simulink model "SF043A_TqOscn"  (R2013b)
settings: Solver=FixedStepDiscrete  SolverMode=SingleTasking  StartTime=0.0  StopTime=1  FixedStep=0.002  RelTol=1e-3
values from neighbouring files (symbols this model uses):
  ARCHGLBPRM_2MILLISEC_SEC_F32 = DataDict.Constant    [SF043A_TqOscn_DataDict.m]
  ARCHGLBPRM_2PI_ULS_F32 = DataDict.Constant    [SF043A_TqOscn_DataDict.m]
  DCTHD_MOTNWTMTR_F32 = DataDict.Constant    [SF043A_TqOscn_DataDict.m]
  DFTFALLRAMPRATE_MOTNWTMTRPERSEC_F32 = DataDict.Constant    [SF043A_TqOscn_DataDict.m]
  DFTPHAAGINC_MATRAD_F32 = DataDict.Constant    [SF043A_TqOscn_DataDict.m]
  DFTRISNGRAMPRATE_MOTNWTMTRPERSEC_F32 = DataDict.Constant    [SF043A_TqOscn_DataDict.m]
  FltInj_f32 = DataDict.Client    [SF043A_TqOscn_DataDict.m]
  FLTINJ_TQOSCN_PREFINALCMD = DataDict.Constant    [SF043A_TqOscn_DataDict.m]
  MAXAMP_MOTNWTMTR_F32 = DataDict.Constant    [SF043A_TqOscn_DataDict.m]
  MAXRAMPRATE_MOTNWTMTR_F32 = DataDict.Constant    [SF043A_TqOscn_DataDict.m]
  MINAMP_MOTNWTMTR_F32 = DataDict.Constant    [SF043A_TqOscn_DataDict.m]
  MINRAMPRATE_MOTNWTMTR_F32 = DataDict.Constant    [SF043A_TqOscn_DataDict.m]
  TqOscnAmpLimY = DataDict.Calibration    [SF043A_TqOscn_DataDict.m]
  TqOscnFallRampRateCal = DataDict.Calibration    [SF043A_TqOscn_DataDict.m]
  TqOscnFrqIn = DataDict.Calibration    [SF043A_TqOscn_DataDict.m]
  TqOscnRisngRampRateCal = DataDict.Calibration    [SF043A_TqOscn_DataDict.m]
  TqOscnUseRampRateCal = DataDict.Calibration    [SF043A_TqOscn_DataDict.m]
libraries: NxtrLim x6, simulink x3, NxtrAbslt x3, Fil x2, FixdToFloat x2, autosarlib x1, NxtrMath x1, FloatToFixd x1
(part 2 of 2)

== system SF043A_TqOscn/TqOscn/TqOscnPer1/Amplitude Rate Limiter/SetToZero ==
  Action Port : ActionPort  ActionType=then
  Constant4 : Constant  Value=0  OutDataTypeStr=single
      settings: AttributesFormatString=%<OutDataTypeStr>
  CopyRight2 : Subsystem  Description=|  mask(Copyright Information){none=on}
      | Copyright info block.                                               
      |                                                                     
      | Place copyright information at the top of every subsystem in design.
      mask prompts: none "No parameters"
      mask help: Place copyright information at the top of every subsystem in design.
      mask Display:
      | NxtrConf = 'Nexteer Confidential';
      | 
      | sys = bdroot; %handle for the current model ("system")
      | first = get_param(sys,'Created');
      | if(isempty(first))
      |     first = datestr(now,'yyyy');
      | else
      |     first = first(end-3:end);  %year is last four digits
      | end
      | 
      | last = get_param(sys,'LastModifiedDate');
      | if isempty(last)
      |     last = datestr(now,'yyyy');
      | else
      |     last = last(end-3:end);
      | end
      | 
      | if strcmp(first,last)
      |     fprintf('%s -- Copyright %s Nexteer',NxtrConf,first)
      | else
      |     fprintf('%s -- %s%s- %s Nexteer',NxtrConf,char(169),first,last)
      | end
  Out1 : Outport
  wires:
  Constant4/1 -> Out1/1

== system SF043A_TqOscn/TqOscn/TqOscnPer1/Amplitude Rate Limiter/UseCals ==
  Action Port : ActionPort  ActionType=then
  Constant1 : Constant  Value=TqOscnRisngRampRateCal
  Constant2 : Constant  Value=TqOscnFallRampRateCal
  CopyRight2 : Subsystem  Description=|  mask(Copyright Information){none=on}
      | Copyright info block.                                               
      |                                                                     
      | Place copyright information at the top of every subsystem in design.
      mask prompts: none "No parameters"
      mask help: Place copyright information at the top of every subsystem in design.
      mask Display:
      | NxtrConf = 'Nexteer Confidential';
      | 
      | sys = bdroot; %handle for the current model ("system")
      | first = get_param(sys,'Created');
      | if(isempty(first))
      |     first = datestr(now,'yyyy');
      | else
      |     first = first(end-3:end);  %year is last four digits
      | end
      | 
      | last = get_param(sys,'LastModifiedDate');
      | if isempty(last)
      |     last = datestr(now,'yyyy');
      | else
      |     last = last(end-3:end);
      | end
      | 
      | if strcmp(first,last)
      |     fprintf('%s -- Copyright %s Nexteer',NxtrConf,first)
      | else
      |     fprintf('%s -- %s%s- %s Nexteer',NxtrConf,char(169),first,last)
      | end
  Out1 : Outport
  Out2 : Outport  Port=2
  wires:
  Constant2/1 -> Out1/1
  Constant1/1 -> Out2/1

== system SF043A_TqOscn/TqOscn/TqOscnPer1/Amplitude Rate Limiter/UseCmd ==
  In1 : Inport
  Action Port : ActionPort  ActionType=else
  Out1 : Outport
  wires:
  In1/1 -> Out1/1

== system SF043A_TqOscn/TqOscn/TqOscnPer1/Amplitude Rate Limiter/UseInputs ==
  In1 : Inport
  In2 : Inport  Port=2
  Action Port : ActionPort  ActionType=else
  Out1 : Outport
  Out2 : Outport  Port=2
  wires:
  In2/1 -> Out2/1
  In1/1 -> Out1/1

== system SF043A_TqOscn/TqOscn/TqOscnPer1/Angle Wrapper/CopyRight2 ==

== system SF043A_TqOscn/TqOscn/TqOscnPer1/Angle Wrapper/Pass_through ==
  In1 : Inport
  Action Port : ActionPort  ActionType=else
  CopyRight2 : Subsystem  Description=|  mask(Copyright Information){none=on}
      | Copyright info block.                                               
      |                                                                     
      | Place copyright information at the top of every subsystem in design.
      mask prompts: none "No parameters"
      mask help: Place copyright information at the top of every subsystem in design.
      mask Display:
      | NxtrConf = 'Nexteer Confidential';
      | 
      | sys = bdroot; %handle for the current model ("system")
      | first = get_param(sys,'Created');
      | if(isempty(first))
      |     first = datestr(now,'yyyy');
      | else
      |     first = first(end-3:end);  %year is last four digits
      | end
      | 
      | last = get_param(sys,'LastModifiedDate');
      | if isempty(last)
      |     last = datestr(now,'yyyy');
      | else
      |     last = last(end-3:end);
      | end
      | 
      | if strcmp(first,last)
      |     fprintf('%s -- Copyright %s Nexteer',NxtrConf,first)
      | else
      |     fprintf('%s -- %s%s- %s Nexteer',NxtrConf,char(169),first,last)
      | end
  Out1 : Outport
  wires:
  In1/1 -> Out1/1

== system SF043A_TqOscn/TqOscn/TqOscnPer1/Angle Wrapper/Subtract_2pi ==
  In1 : Inport
  Action Port : ActionPort  ActionType=then
  Constant : Constant  Value=ARCHGLBPRM_2PI_ULS_F32
  CopyRight2 : Subsystem  Description=|  mask(Copyright Information){none=on}
      | Copyright info block.                                               
      |                                                                     
      | Place copyright information at the top of every subsystem in design.
      mask prompts: none "No parameters"
      mask help: Place copyright information at the top of every subsystem in design.
      mask Display:
      | NxtrConf = 'Nexteer Confidential';
      | 
      | sys = bdroot; %handle for the current model ("system")
      | first = get_param(sys,'Created');
      | if(isempty(first))
      |     first = datestr(now,'yyyy');
      | else
      |     first = first(end-3:end);  %year is last four digits
      | end
      | 
      | last = get_param(sys,'LastModifiedDate');
      | if isempty(last)
      |     last = datestr(now,'yyyy');
      | else
      |     last = last(end-3:end);
      | end
      | 
      | if strcmp(first,last)
      |     fprintf('%s -- Copyright %s Nexteer',NxtrConf,first)
      | else
      |     fprintf('%s -- %s%s- %s Nexteer',NxtrConf,char(169),first,last)
      | end
  Subtract : Sum  Inputs=+-
  Out1 : Outport
  wires:
  In1/1 -> Subtract/1
  Subtract/1 -> Out1/1
  Constant/1 -> Subtract/2

== system SF043A_TqOscn/TqOscn/TqOscnPer1/CheckFlag/CopyRight2 ==

== system SF043A_TqOscn/TqOscn/TqOscnPer1/CheckFlag/SetToZero ==
  Action Port : ActionPort  ActionType=else
  Constant2 : Constant  Value=0  OutDataTypeStr=single
      settings: AttributesFormatString=%<OutDataTypeStr>
  CopyRight2 : Subsystem  Description=|  mask(Copyright Information){none=on}
      | Copyright info block.                                               
      |                                                                     
      | Place copyright information at the top of every subsystem in design.
      mask prompts: none "No parameters"
      mask help: Place copyright information at the top of every subsystem in design.
      mask Display:
      | NxtrConf = 'Nexteer Confidential';
      | 
      | sys = bdroot; %handle for the current model ("system")
      | first = get_param(sys,'Created');
      | if(isempty(first))
      |     first = datestr(now,'yyyy');
      | else
      |     first = first(end-3:end);  %year is last four digits
      | end
      | 
      | last = get_param(sys,'LastModifiedDate');
      | if isempty(last)
      |     last = datestr(now,'yyyy');
      | else
      |     last = last(end-3:end);
      | end
      | 
      | if strcmp(first,last)
      |     fprintf('%s -- Copyright %s Nexteer',NxtrConf,first)
      | else
      |     fprintf('%s -- %s%s- %s Nexteer',NxtrConf,char(169),first,last)
      | end
  Out1 : Outport
  wires:
  Constant2/1 -> Out1/1

== system SF043A_TqOscn/TqOscn/TqOscnPer1/CheckFlag/UseInput ==
  In1 : Inport
  Action Port : ActionPort  ActionType=then
  CopyRight2 : Subsystem  Description=|  mask(Copyright Information){none=on}
      | Copyright info block.                                               
      |                                                                     
      | Place copyright information at the top of every subsystem in design.
      mask prompts: none "No parameters"
      mask help: Place copyright information at the top of every subsystem in design.
      mask Display:
      | NxtrConf = 'Nexteer Confidential';
      | 
      | sys = bdroot; %handle for the current model ("system")
      | first = get_param(sys,'Created');
      | if(isempty(first))
      |     first = datestr(now,'yyyy');
      | else
      |     first = first(end-3:end);  %year is last four digits
      | end
      | 
      | last = get_param(sys,'LastModifiedDate');
      | if isempty(last)
      |     last = datestr(now,'yyyy');
      | else
      |     last = last(end-3:end);
      | end
      | 
      | if strcmp(first,last)
      |     fprintf('%s -- Copyright %s Nexteer',NxtrConf,first)
      | else
      |     fprintf('%s -- %s%s- %s Nexteer',NxtrConf,char(169),first,last)
      | end
  Out1 : Outport
  wires:
  In1/1 -> Out1/1

== system SF043A_TqOscn/TqOscn/TqOscnPer1/DC Check/CopyRight2 ==

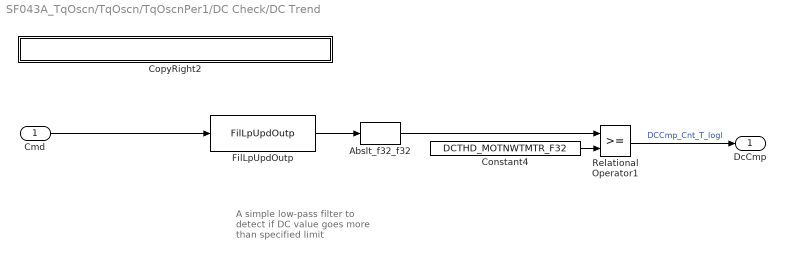
== system SF043A_TqOscn/TqOscn/TqOscnPer1/DC Check/DC Trend ==
  note: A simple low-pass filter to detect if DC value goes more than specified limit
  Cmd : Inport
  Abslt_f32_f32 : NxtrAbslt/Abslt_f32_f32  SFunctionSpec=single y1 = Abslt_f32_f32(single u1)
      settings: AttributesFormatString=%<Name>
  Constant4 : Constant  RequirementInfo={'linktype_rmi_doors' '0000a558 (/E-STEER Core/SubSystem Specifications/Application Functions/SF043A Torque Oscillation)' '#SF043A_335' 'true' 'REQ:SF043A_335' '' } %GIDa_6c203f5b_5b38_493c_a4ae_d80a5c53087b  Value=DCTHD_MOTNWTMTR_F32
  CopyRight2 : Subsystem  Description=|  mask(Copyright Information){none=on}
      | Copyright info block.                                               
      |                                                                     
      | Place copyright information at the top of every subsystem in design.
      mask prompts: none "No parameters"
      mask help: Place copyright information at the top of every subsystem in design.
      mask Display:
      | NxtrConf = 'Nexteer Confidential';
      | 
      | sys = bdroot; %handle for the current model ("system")
      | first = get_param(sys,'Created');
      | if(isempty(first))
      |     first = datestr(now,'yyyy');
      | else
      |     first = first(end-3:end);  %year is last four digits
      | end
      | 
      | last = get_param(sys,'LastModifiedDate');
      | if isempty(last)
      |     last = datestr(now,'yyyy');
      | else
      |     last = last(end-3:end);
      | end
      | 
      | if strcmp(first,last)
      |     fprintf('%s -- Copyright %s Nexteer',NxtrConf,first)
      | else
      |     fprintf('%s -- %s%s- %s Nexteer',NxtrConf,char(169),first,last)
      | end
  FilLpUpdOutp : Fil/FilLpUpdOutp  RequirementInfo={'linktype_rmi_doors' '0000a558 (/E-STEER Core/SubSystem Specifications/Application Functions/SF043A Torque Oscillation)' '#SF043A_334' 'true' 'REQ:SF043A_334' '' } %GIDa_7480e813_7b8e_4b56_a323_4ea049146c63  StVar=PreFinalCmdLpFil
      settings: AttributesFormatString=StVar: %<StVar>
  Relational Operator1 : RelationalOperator  RequirementInfo={'linktype_rmi_doors' '0000a558 (/E-STEER Core/SubSystem Specifications/Application Functions/SF043A Torque Oscillation)' '#SF043A_335' 'true' 'REQ:SF043A_335' '' } %GIDa_618fbe93_81fb_4f23_8b51_b3d5bed42e02  OutDataTypeStr=boolean
  DcCmp : Outport  RequirementInfo={'linktype_rmi_doors' '0000a558 (/E-STEER Core/SubSystem Specifications/Application Functions/SF043A Torque Oscillation)' '#SF043A_335' 'true' 'REQ:SF043A_335' '' } %GIDa_1afcdcae_25d3_461d_aaa1_98d84ed6aaf2
  wires:
  FilLpUpdOutp/1 -> Abslt_f32_f32/1
  Constant4/1 -> Relational Operator1/2
  Relational Operator1/1 -> DcCmp/1  "DCCmp_Cnt_T_logl"
  Abslt_f32_f32/1 -> Relational Operator1/1
  Cmd/1 -> FilLpUpdOutp/1

== system SF043A_TqOscn/TqOscn/TqOscnPer1/DC Check/DC_Detd ==
  Action Port : ActionPort  ActionType=then
  Constant : Constant  Value=0  OutDataTypeStr=single
      settings: AttributesFormatString=%<OutDataTypeStr>
  Constant1 : Constant  Value=true  OutDataTypeStr=boolean
      settings: AttributesFormatString=%<OutDataTypeStr>
  CopyRight2 : Subsystem  Description=|  mask(Copyright Information){none=on}
      | Copyright info block.                                               
      |                                                                     
      | Place copyright information at the top of every subsystem in design.
      mask prompts: none "No parameters"
      mask help: Place copyright information at the top of every subsystem in design.
      mask Display:
      | NxtrConf = 'Nexteer Confidential';
      | 
      | sys = bdroot; %handle for the current model ("system")
      | first = get_param(sys,'Created');
      | if(isempty(first))
      |     first = datestr(now,'yyyy');
      | else
      |     first = first(end-3:end);  %year is last four digits
      | end
      | 
      | last = get_param(sys,'LastModifiedDate');
      | if isempty(last)
      |     last = datestr(now,'yyyy');
      | else
      |     last = last(end-3:end);
      | end
      | 
      | if strcmp(first,last)
      |     fprintf('%s -- Copyright %s Nexteer',NxtrConf,first)
      | else
      |     fprintf('%s -- %s%s- %s Nexteer',NxtrConf,char(169),first,last)
      | end
  Cmd : Outport
  Excdd : Outport  Port=2
  wires:
  Constant/1 -> Cmd/1
  Constant1/1 -> Excdd/1

== system SF043A_TqOscn/TqOscn/TqOscnPer1/DC Check/DC_ok ==
  In1 : Inport
  Action Port : ActionPort  ActionType=else
  Constant1 : Constant  Value=false  OutDataTypeStr=boolean
      settings: AttributesFormatString=%<OutDataTypeStr>
  CopyRight2 : Subsystem  Description=|  mask(Copyright Information){none=on}
      | Copyright info block.                                               
      |                                                                     
      | Place copyright information at the top of every subsystem in design.
      mask prompts: none "No parameters"
      mask help: Place copyright information at the top of every subsystem in design.
      mask Display:
      | NxtrConf = 'Nexteer Confidential';
      | 
      | sys = bdroot; %handle for the current model ("system")
      | first = get_param(sys,'Created');
      | if(isempty(first))
      |     first = datestr(now,'yyyy');
      | else
      |     first = first(end-3:end);  %year is last four digits
      | end
      | 
      | last = get_param(sys,'LastModifiedDate');
      | if isempty(last)
      |     last = datestr(now,'yyyy');
      | else
      |     last = last(end-3:end);
      | end
      | 
      | if strcmp(first,last)
      |     fprintf('%s -- Copyright %s Nexteer',NxtrConf,first)
      | else
      |     fprintf('%s -- %s%s- %s Nexteer',NxtrConf,char(169),first,last)
      | end
  Cmd : Outport
  Excdd : Outport  Port=2
  wires:
  In1/1 -> Cmd/1
  Constant1/1 -> Excdd/1

== system SF043A_TqOscn/TqOscn/TqOscnPer1/FltInj_f32 client/CodeGen ==
  note: NOTE 1:  Simulink 2013b cannot handle InOut arguments, so the operation
      |                 prototype inside this block is not quite right.
      |
      | NOTE 2:  Do not use this variant for simulation.  Sig_Out = zero, always.
  note: FltInj_f32(float32 *SigPah, uint16 LocnKey)
  Sig : Inport
  "LocnKey  " : Inport  Port=2
  CopyRight1 : Subsystem  Description=|  mask(Copyright Information){none=on}
      | Copyright info block.                                               
      |                                                                     
      | Place copyright information at the top of every subsystem in design.
      mask prompts: none "No parameters"
      mask help: Place copyright information at the top of every subsystem in design.
      mask Display:
      | NxtrConf = 'Nexteer Confidential';
      | 
      | sys = bdroot; %handle for the current model ("system")
      | first = get_param(sys,'Created');
      | if(isempty(first))
      |     first = datestr(now,'yyyy');
      | else
      |     first = first(end-3:end);  %year is last four digits
      | end
      | 
      | last = get_param(sys,'LastModifiedDate');
      | if isempty(last)
      |     last = datestr(now,'yyyy');
      | else
      |     last = last(end-3:end);
      | end
      | 
      | if strcmp(first,last)
      |     fprintf('%s -- Copyright %s Nexteer',NxtrConf,first)
      | else
      |     fprintf('%s -- %s%s- %s Nexteer',NxtrConf,char(169),first,last)
      | end
  Invoke AUTOSAR Server Operation : autosarlib/Invoke AUTOSAR Server Operation  portName=FltInj_f32  operationPrototype=FltInj_f32(IN single SigPah_ArgIn, OUT single SigPah_ArgOut, IN uint16 LocnKey)  interfacePath=/AUTOSAR/Interface  serverType=Application software  showErrorStatus=off  SAMPLETIME=-1  showARPortLabels=on
  Sig_Out : Outport  OutDataTypeStr=single
  wires:
  Sig/1 -> Invoke AUTOSAR Server Operation/1
  "LocnKey  "/1 -> Invoke AUTOSAR Server Operation/2
  Invoke AUTOSAR Server Operation/1 -> Sig_Out/1

== system SF043A_TqOscn/TqOscn/TqOscnPer1/FltInj_f32 client/CopyRight1 ==

== system SF043A_TqOscn/TqOscn/TqOscnPer1/FltInj_f32 client/Sim ==
  note: This block requires no modification by FDD author.
      |
      | This block does not actually simulate any fault injection.  It is simply a pass-thru.
      |
      | Input port (#2) simply terminates its signal, but we are trying to force the FDD author
      | to properly use the FltInjectionLocType enumeration in FDD model.
  note: EA4.x Fault Injection
  Sig : Inport
  "LocnKey  " : Inport  Port=2  OutDataTypeStr=uint16
  CopyRight1 : Subsystem  Description=|  mask(Copyright Information){none=on}
      | Copyright info block.                                               
      |                                                                     
      | Place copyright information at the top of every subsystem in design.
      mask prompts: none "No parameters"
      mask help: Place copyright information at the top of every subsystem in design.
      mask Display:
      | NxtrConf = 'Nexteer Confidential';
      | 
      | sys = bdroot; %handle for the current model ("system")
      | first = get_param(sys,'Created');
      | if(isempty(first))
      |     first = datestr(now,'yyyy');
      | else
      |     first = first(end-3:end);  %year is last four digits
      | end
      | 
      | last = get_param(sys,'LastModifiedDate');
      | if isempty(last)
      |     last = datestr(now,'yyyy');
      | else
      |     last = last(end-3:end);
      | end
      | 
      | if strcmp(first,last)
      |     fprintf('%s -- Copyright %s Nexteer',NxtrConf,first)
      | else
      |     fprintf('%s -- %s%s- %s Nexteer',NxtrConf,char(169),first,last)
      | end
  Terminator : Terminator
  Sig_Out : Outport
  wires:
  Sig/1 -> Sig_Out/1
  "LocnKey  "/1 -> Terminator/1

== system SF043A_TqOscn/TqOscn/TqOscnPer1/Set_false/CopyRight2 ==

== system SF043A_TqOscn/TqOscn/TqOscnPer1/Set_true/CopyRight2 ==

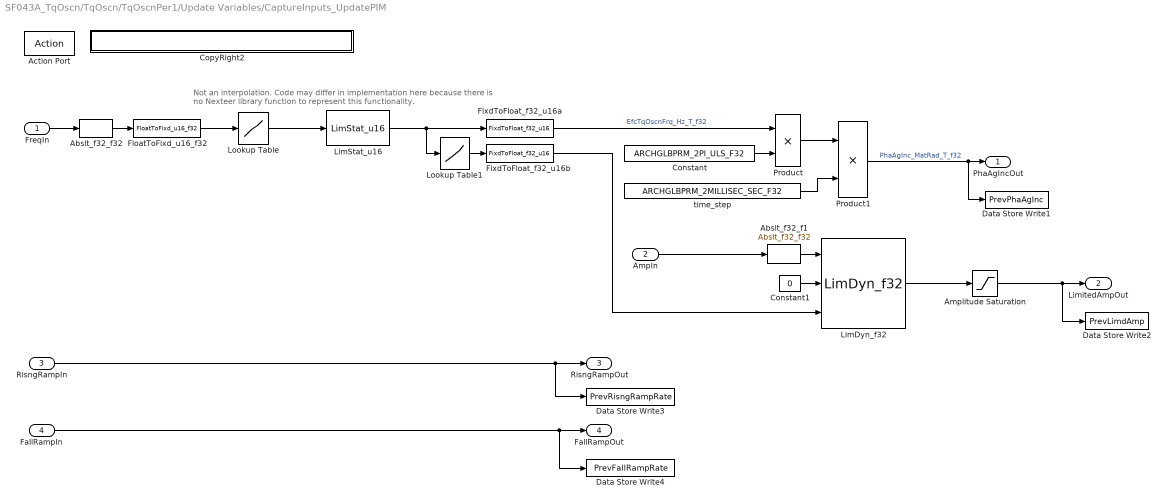
== system SF043A_TqOscn/TqOscn/TqOscnPer1/Update Variables/CaptureInputs_UpdatePIM ==
  note: Not an interpolation.  Code may differ in implementation here because there
      | is no Nexteer library function to represent this functionality.
  FreqIn : Inport  RequirementInfo={} %GIDa_1e1cd702_07fe_49fe_8947_31431a58e45b
  AmpIn : Inport  RequirementInfo={'linktype_rmi_doors' '0000a558 (/E-STEER Core/SubSystem Specifications/Application Functions/SF043A Torque Oscillation)' '#SF043A_320' 'true' 'REQ:SF043A_320' '' } %GIDa_8088d360_8b23_47d1_855a_eb1de7ebd5e4  Port=2
  RisngRampIn : Inport  RequirementInfo={'linktype_rmi_doors' '0000a558 (/E-STEER Core/SubSystem Specifications/Application Functions/SF043A Torque Oscillation)' '#SF043A_321' 'true' 'REQ:SF043A_321' '' } %GIDa_b7d07da4_db6a_4e3d_9af0_8782b4d0f024  Port=3
  FallRampIn : Inport  RequirementInfo={'linktype_rmi_doors' '0000a558 (/E-STEER Core/SubSystem Specifications/Application Functions/SF043A Torque Oscillation)' '#SF043A_322' 'true' 'REQ:SF043A_322' '' } %GIDa_962124a2_4b93_46f5_ace1_33638640915d  Port=4
  Action Port : ActionPort  ActionType=then
  Abslt_f32_f1 : NxtrAbslt/Abslt_f32_f32  RequirementInfo={'linktype_rmi_doors' '0000a558 (/E-STEER Core/SubSystem Specifications/Application Functions/SF043A Torque Oscillation)' '#SF043A_320' 'true' 'REQ:SF043A_320' '' } %GIDa_686dcb48_c1ec_4c2a_924a_e657627dc353  SFunctionSpec=single y1 = Abslt_f32_f32(single u1)
      settings: AttributesFormatString=%<Name>
  Abslt_f32_f32 : NxtrAbslt/Abslt_f32_f32  RequirementInfo={} %GIDa_20961518_0603_4677_bd06_aafd74fe8b47  SFunctionSpec=single y1 = Abslt_f32_f32(single u1)
      settings: AttributesFormatString=%<Name>
  Amplitude Saturation : Saturate  RequirementInfo={'linktype_rmi_doors' '0000a558 (/E-STEER Core/SubSystem Specifications/Application Functions/SF043A Torque Oscillation)' '#SF043A_320' 'true' 'REQ:SF043A_320' '' ; 'linktype_rmi_doors' '0000a558 (/E-STEER Core/SubSystem Specifications/Application Functions/SF043A Torque Oscillation)' '#SF043A_323' 'true' 'REQ:SF043A_323' '' } %GIDa_b14632e0_b3b4_4b21_aab6_08b820319b05  UpperLimit=MAXAMP_MOTNWTMTR_F32  LowerLimit=MINAMP_MOTNWTMTR_F32
      settings: AttributesFormatString=UPR=%<UpperLimit>\nLWR=%<LowerLimit>
  Constant : Constant  Value=ARCHGLBPRM_2PI_ULS_F32
  Constant1 : Constant  RequirementInfo={'linktype_rmi_doors' '0000a558 (/E-STEER Core/SubSystem Specifications/Application Functions/SF043A Torque Oscillation)' '#SF043A_320' 'true' 'REQ:SF043A_320' '' } %GIDa_c355547a_ffc8_4f22_aa5f_e81363987f9d  Value=0  OutDataTypeStr=single
      settings: AttributesFormatString=%<OutDataTypeStr>
  CopyRight2 : Subsystem  Description=|  mask(Copyright Information){none=on}
      | Copyright info block.                                               
      |                                                                     
      | Place copyright information at the top of every subsystem in design.
      mask prompts: none "No parameters"
      mask help: Place copyright information at the top of every subsystem in design.
      mask Display:
      | NxtrConf = 'Nexteer Confidential';
      | 
      | sys = bdroot; %handle for the current model ("system")
      | first = get_param(sys,'Created');
      | if(isempty(first))
      |     first = datestr(now,'yyyy');
      | else
      |     first = first(end-3:end);  %year is last four digits
      | end
      | 
      | last = get_param(sys,'LastModifiedDate');
      | if isempty(last)
      |     last = datestr(now,'yyyy');
      | else
      |     last = last(end-3:end);
      | end
      | 
      | if strcmp(first,last)
      |     fprintf('%s -- Copyright %s Nexteer',NxtrConf,first)
      | else
      |     fprintf('%s -- %s%s- %s Nexteer',NxtrConf,char(169),first,last)
      | end
  Data Store Write1 : DataStoreWrite  DataStoreName=PrevPhaAgInc
  Data Store Write2 : DataStoreWrite  RequirementInfo={'linktype_rmi_doors' '0000a558 (/E-STEER Core/SubSystem Specifications/Application Functions/SF043A Torque Oscillation)' '#SF043A_320' 'true' 'REQ:SF043A_320' '' } %GIDa_684092d3_0e9c_4b10_90ad_6b2ae104cb4a  DataStoreName=PrevLimdAmp
  Data Store Write3 : DataStoreWrite  RequirementInfo={'linktype_rmi_doors' '0000a558 (/E-STEER Core/SubSystem Specifications/Application Functions/SF043A Torque Oscillation)' '#SF043A_321' 'true' 'REQ:SF043A_321' '' } %GIDa_a20425e6_b584_439e_a32a_f492801bed71  DataStoreName=PrevRisngRampRate
  Data Store Write4 : DataStoreWrite  RequirementInfo={'linktype_rmi_doors' '0000a558 (/E-STEER Core/SubSystem Specifications/Application Functions/SF043A Torque Oscillation)' '#SF043A_322' 'true' 'REQ:SF043A_322' '' } %GIDa_8daa8598_b3f2_434a_b3dd_69d33c4d5e6c  DataStoreName=PrevFallRampRate
  FixdToFloat_f32_u16a : FixdToFloat/FixdToFloat_f32_u16  Param1=8
  FixdToFloat_f32_u16b : FixdToFloat/FixdToFloat_f32_u16  Param1=11
  FloatToFixd_u16_f32 : FloatToFixd/FloatToFixd_u16_f32  RequirementInfo={} %GIDa_ab6b0326_8659_495f_9d5e_ae96f25dc97e  Param1=8
  LimDyn_f32 : NxtrLim/LimDyn_f32  RequirementInfo={'linktype_rmi_doors' '0000a558 (/E-STEER Core/SubSystem Specifications/Application Functions/SF043A Torque Oscillation)' '#SF043A_320' 'true' 'REQ:SF043A_320' '' } %GIDa_6df0978f_0905_4878_80b3_8930e7448859
  LimStat_u16 : NxtrLim/LimStat_u16  RequirementInfo={'linktype_rmi_doors' '0000a558 (/E-STEER Core/SubSystem Specifications/Application Functions/SF043A Torque Oscillation)' '#SF043A_315' 'true' 'REQ:SF043A_315' '' } %GIDa_3eeeaba6_26b8_4e57_99e8_6c115ad5e6c8  LoLim=MINFRQ_CNT_U16  HiLim=MAXFRQ_CNT_U16
      settings: AttributesFormatString=|
      | Low Limit: %<LoLim>
      | High Limit:%<HiLim>
  Lookup Table : Lookup  RequirementInfo={'linktype_rmi_doors' '0000a558 (/E-STEER Core/SubSystem Specifications/Application Functions/SF043A Torque Oscillation)' '#SF043A_316' 'true' 'REQ:SF043A_316' '' ; 'linktype_rmi_doors' '0000a558 (/E-STEER Core/SubSystem Specifications/Application Functions/SF043A Torque Oscillation)' '#SF043A_317' 'true' 'REQ:SF043A_317' '' ; 'linktype_rmi_doors' '0000a558 (/E-STEER Core/SubSystem Specifications/Application Functions/SF043A Torque Oscillation)' '#SF043A_318' 'true' 'REQ:SF043A_318' '' } %GIDa_2a87b88c_2148_4626_8153_3d00cbb05ac0  InputValues=TqOscnFrqIn  Table=TqOscnFrqIn  LookUpMeth=Use Input Below
      settings: AttributesFormatString=Input=%<InputValues>\nOutput=%<OutputValues>\nLookup Method=\n%<LookUpMeth>
  Lookup Table1 : Lookup  RequirementInfo={'linktype_rmi_doors' '0000a558 (/E-STEER Core/SubSystem Specifications/Application Functions/SF043A Torque Oscillation)' '#SF043A_324' 'true' 'REQ:SF043A_324' '' } %GIDa_13f9bc77_c553_4d5c_8f17_4791133e4b15  InputValues=TqOscnFrqIn  Table=TqOscnAmpLimY  LookUpMeth=Use Input Below
      settings: AttributesFormatString=Input=%<InputValues>\nOutput=%<OutputValues>\nLookup Method=\n%<LookUpMeth>
  Product : Product  RndMeth=Zero
  Product1 : Product  RndMeth=Zero
  time_step : Constant  Value=ARCHGLBPRM_2MILLISEC_SEC_F32
  PhaAgIncOut : Outport
  LimitedAmpOut : Outport  RequirementInfo={'linktype_rmi_doors' '0000a558 (/E-STEER Core/SubSystem Specifications/Application Functions/SF043A Torque Oscillation)' '#SF043A_320' 'true' 'REQ:SF043A_320' '' } %GIDa_feed8225_5bb0_4298_b6e6_992887f1e478  Port=2
  RisngRampOut : Outport  RequirementInfo={'linktype_rmi_doors' '0000a558 (/E-STEER Core/SubSystem Specifications/Application Functions/SF043A Torque Oscillation)' '#SF043A_321' 'true' 'REQ:SF043A_321' '' } %GIDa_b10902d9_9d3b_44d9_b725_798dc8615d28  Port=3
  FallRampOut : Outport  RequirementInfo={'linktype_rmi_doors' '0000a558 (/E-STEER Core/SubSystem Specifications/Application Functions/SF043A Torque Oscillation)' '#SF043A_322' 'true' 'REQ:SF043A_322' '' } %GIDa_aa2544d0_c17f_4ce5_be5d_55bb8d958bae  Port=4
  wires:
  AmpIn/1 -> Abslt_f32_f1/1
  Lookup Table/1 -> LimStat_u16/1
  LimStat_u16/1 -> FixdToFloat_f32_u16a/1, Lookup Table1/1
  Product/1 -> Product1/1
  time_step/1 -> Product1/2
  LimDyn_f32/1 -> Amplitude Saturation/1
  FreqIn/1 -> Abslt_f32_f32/1
  Lookup Table1/1 -> FixdToFloat_f32_u16b/1
  Constant/1 -> Product/2
  Abslt_f32_f1/1 -> LimDyn_f32/1
  Abslt_f32_f32/1 -> FloatToFixd_u16_f32/1
  Amplitude Saturation/1 -> Data Store Write2/1, LimitedAmpOut/1
  Product1/1 -> Data Store Write1/1, PhaAgIncOut/1  "PhaAgInc_MatRad_T_f32"
  FallRampIn/1 -> Data Store Write4/1, FallRampOut/1
  Constant1/1 -> LimDyn_f32/2
  RisngRampIn/1 -> Data Store Write3/1, RisngRampOut/1
  FloatToFixd_u16_f32/1 -> Lookup Table/1
  FixdToFloat_f32_u16a/1 -> Product/1  "EfcTqOscnFrq_Hz_T_f32"
  FixdToFloat_f32_u16b/1 -> LimDyn_f32/3

== system SF043A_TqOscn/TqOscn/TqOscnPer1/Update Variables/CopyRight2 ==

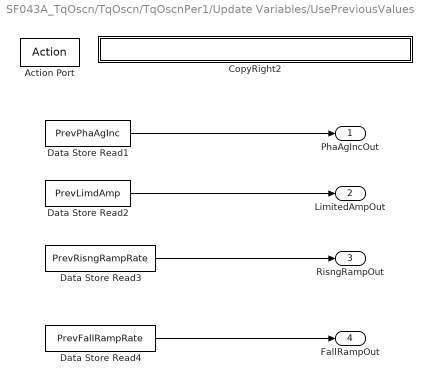
== system SF043A_TqOscn/TqOscn/TqOscnPer1/Update Variables/UsePreviousValues ==
  Action Port : ActionPort  ActionType=else
  CopyRight2 : Subsystem  Description=|  mask(Copyright Information){none=on}
      | Copyright info block.                                               
      |                                                                     
      | Place copyright information at the top of every subsystem in design.
      mask prompts: none "No parameters"
      mask help: Place copyright information at the top of every subsystem in design.
      mask Display:
      | NxtrConf = 'Nexteer Confidential';
      | 
      | sys = bdroot; %handle for the current model ("system")
      | first = get_param(sys,'Created');
      | if(isempty(first))
      |     first = datestr(now,'yyyy');
      | else
      |     first = first(end-3:end);  %year is last four digits
      | end
      | 
      | last = get_param(sys,'LastModifiedDate');
      | if isempty(last)
      |     last = datestr(now,'yyyy');
      | else
      |     last = last(end-3:end);
      | end
      | 
      | if strcmp(first,last)
      |     fprintf('%s -- Copyright %s Nexteer',NxtrConf,first)
      | else
      |     fprintf('%s -- %s%s- %s Nexteer',NxtrConf,char(169),first,last)
      | end
  Data Store Read1 : DataStoreRead  DataStoreName=PrevPhaAgInc
  Data Store Read2 : DataStoreRead  DataStoreName=PrevLimdAmp
  Data Store Read3 : DataStoreRead  DataStoreName=PrevRisngRampRate
  Data Store Read4 : DataStoreRead  DataStoreName=PrevFallRampRate
  PhaAgIncOut : Outport
  LimitedAmpOut : Outport  Port=2
  RisngRampOut : Outport  Port=3
  FallRampOut : Outport  Port=4
  wires:
  Data Store Read4/1 -> FallRampOut/1
  Data Store Read3/1 -> RisngRampOut/1
  Data Store Read1/1 -> PhaAgIncOut/1
  Data Store Read2/1 -> LimitedAmpOut/1

== system SF043A_TqOscn/TqOscn/TqOscnPer1/Amplitude Rate Limiter/SetToZero/CopyRight2 ==

== system SF043A_TqOscn/TqOscn/TqOscnPer1/Amplitude Rate Limiter/UseCals/CopyRight2 ==

== system SF043A_TqOscn/TqOscn/TqOscnPer1/Angle Wrapper/Pass_through/CopyRight2 ==

== system SF043A_TqOscn/TqOscn/TqOscnPer1/Angle Wrapper/Subtract_2pi/CopyRight2 ==

== system SF043A_TqOscn/TqOscn/TqOscnPer1/CheckFlag/SetToZero/CopyRight2 ==

== system SF043A_TqOscn/TqOscn/TqOscnPer1/CheckFlag/UseInput/CopyRight2 ==

== system SF043A_TqOscn/TqOscn/TqOscnPer1/DC Check/DC Trend/CopyRight2 ==

== system SF043A_TqOscn/TqOscn/TqOscnPer1/DC Check/DC_Detd/CopyRight2 ==

== system SF043A_TqOscn/TqOscn/TqOscnPer1/DC Check/DC_ok/CopyRight2 ==

== system SF043A_TqOscn/TqOscn/TqOscnPer1/FltInj_f32 client/CodeGen/CopyRight1 ==

== system SF043A_TqOscn/TqOscn/TqOscnPer1/FltInj_f32 client/Sim/CopyRight1 ==

== system SF043A_TqOscn/TqOscn/TqOscnPer1/Update Variables/CaptureInputs_UpdatePIM/CopyRight2 ==

== system SF043A_TqOscn/TqOscn/TqOscnPer1/Update Variables/UsePreviousValues/CopyRight2 ==
